simulink model "cic_rev1"  (R2016a)
settings: Solver=VariableStepAuto  StartTime=0.0  StopTime=10.0  RelTol=1e-3
libraries: components x6, dspsrcs4 x1
settings Model: Creator=noah.huesser  LastModifiedBy=noah.huesser

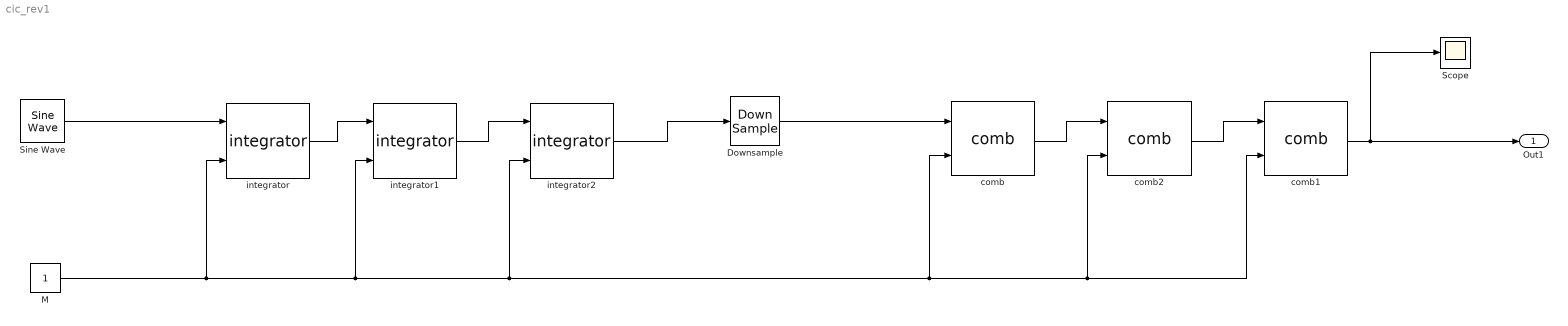
== system cic_rev1 ==
  Downsample : DownSample  N=5
  M : Constant
  Scope : Scope
  Sine Wave : dspsrcs4/Sine Wave  Amplitude=1  Frequency=100  Phase=0  SampleMode=Discrete  OutComplex=Real  CompMethod=Trigonometric fcn  TableSize=Speed  SampleTime=1/1000  SamplesPerFrame=1  ResetState=Restart at time zero  OutputFrames=off  dataType=double  wordLen=16  udDataType=sfix(16)  fracBitsMode=Best precision  numFracBits=15  OutDataTypeStr=double  LastOutDataTypeStr=double
  comb : components/comb
  comb1 : components/comb
  comb2 : components/comb
  integrator : components/integrator
  integrator1 : components/integrator
  integrator2 : components/integrator
  Out1 : Outport
  wires:
  comb/1 -> comb2/1
  integrator1/1 -> integrator2/1
  integrator/1 -> integrator1/1
  comb2/1 -> comb1/1
  comb1/1 -> Scope/1, Out1/1
  M/1 -> comb1/2, comb2/2, comb/2, integrator2/2, integrator1/2, integrator/2
  Downsample/1 -> comb/1
  Sine Wave/1 -> integrator/1
  integrator2/1 -> Downsample/1
